simulink model "RL_FA_system_5ESD0"  (R2021b)
settings: Solver=VariableStepAuto  StartTime=0.0  StopTime=10.0  RelTol=1e-3
values from neighbouring files (symbols this model uses):
  b = 1*10.^-5    (= 1e-05)    [condesign.m]    (also in controller.mat)
  d = 3.125*10.^-5    (= 3.125e-05)    [condesign.m]    (also in controller.mat)
  J1 = 5.8198*10.^-6    (= 5.8198e-06)    [condesign.m]    (also in controller.mat)
  J2 = 4.769*10.^-6    (= 4.769e-06)    [condesign.m]    (also in controller.mat)
  k = 0.2656    [condesign.m]    (also in controller.mat)
  Km = 4.4*10.^-2    (= 0.044)    [condesign.m]    (also in controller.mat)
libraries: cstblocks x2
settings Model: Creator=whendrix  LastModifiedBy=s164604
settings SolverCC: AlgebraicLoopSolver=TrustRegion
settings DebuggingCC: SFMachineParentedDataDiag=warning

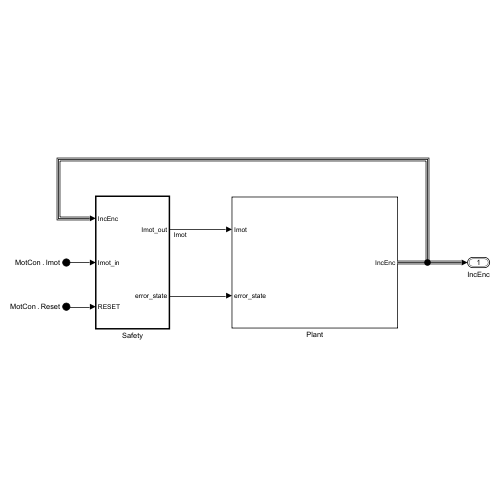
[thumbnail: Simulink's stored preview of the top-level diagram]
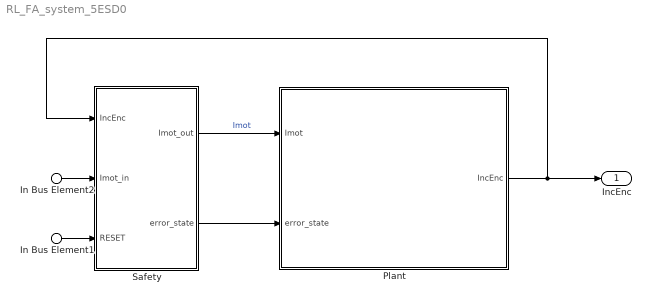
== system RL_FA_system_5ESD0 ==
  In Bus Element2 : Inport  PortName=MotCon  Element=Imot
  In Bus Element1 : Inport  PortName=MotCon  Element=Reset
  Plant : Subsystem
  Safety : Subsystem  TreatAsAtomicUnit=on
  IncEnc : Outport  OutDataTypeStr=Bus: IncEnc
  wires:
  Safety/1(Imot_out) -> Plant/1(Imot)  "Imot"
  In Bus Element2/1 -> Safety/2(Imot_in)
  In Bus Element1/1 -> Safety/3(RESET)
  Plant/1(IncEnc) -> IncEnc/1, Safety/1(IncEnc)
  Safety/2(error_state) -> Plant/2(error_state)

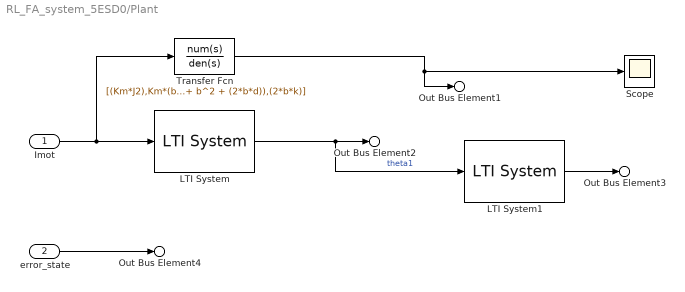
== system RL_FA_system_5ESD0/Plant ==
  Imot : Inport
  error_state : Inport  Port=2
  LTI System : cstblocks/LTI System  sys=G  IC=[]
  LTI System1 : cstblocks/LTI System  sys=G2  IC=[]
  Scope : Scope
  Transfer Fcn : TransferFcn  Numerator=[(Km*J2),Km*(b+d),(Km*k)]  Denominator=[(J1*J2),(J1+J2)*(d+b),((J1+J2)*k + b^2 + (2*b*d)),(2*b*k)]
  Out Bus Element4 : Outport  PortName=IncEnc  Element=error_state
  Out Bus Element2 : Outport  PortName=IncEnc  Element=theta1
  Out Bus Element1 : Outport  PortName=IncEnc  Element=omega1
  Out Bus Element3 : Outport  PortName=IncEnc  Element=theta2
  wires:
  LTI System/1 -> LTI System1/1, Out Bus Element2/1  "theta1"
  LTI System1/1 -> Out Bus Element3/1
  error_state/1 -> Out Bus Element4/1
  Imot/1 -> Transfer Fcn/1, LTI System/1
  Transfer Fcn/1 -> Scope/1, Out Bus Element1/1

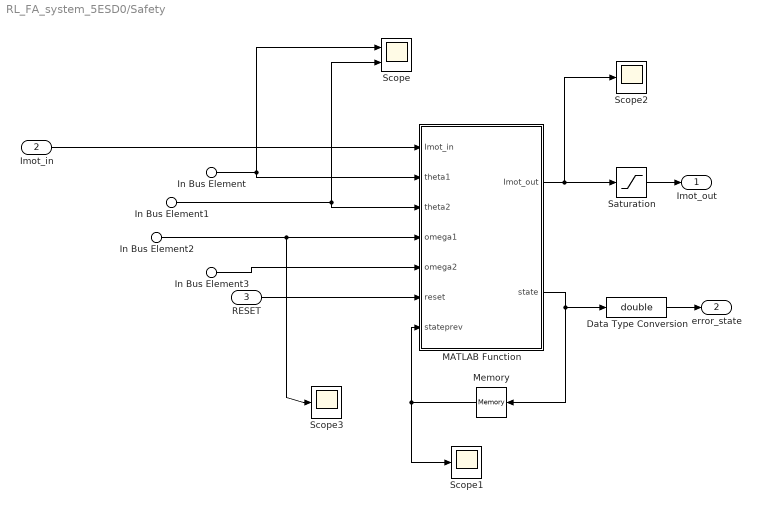
== system RL_FA_system_5ESD0/Safety ==
  In Bus Element : Inport  PortName=IncEnc  Element=theta1
  In Bus Element2 : Inport  PortName=IncEnc  Element=omega1
  In Bus Element1 : Inport  PortName=IncEnc  Element=theta2
  In Bus Element3 : Inport  PortName=IncEnc  Element=omega2
  Imot_in : Inport  Port=2
  RESET : Inport  Port=3
  Data Type Conversion : DataTypeConversion  OutDataTypeStr=double
  MATLAB Function : MATLAB Function  TreatAsAtomicUnit=on
  Memory : Memory
  Saturation : Saturate  UpperLimit=1.83  LowerLimit=-1.83
  Scope : Scope  NumInputPorts=2
  Scope1 : Scope
  Scope2 : Scope
  Scope3 : Scope
  Imot_out : Outport
  error_state : Outport  Port=2
  wires:
  Imot_in/1 -> MATLAB Function/1(Imot_in)
  MATLAB Function/1(Imot_out) -> Scope2/1, Saturation/1
  RESET/1 -> MATLAB Function/6(reset)
  In Bus Element/1 -> Scope/1, MATLAB Function/2(theta1)
  In Bus Element1/1 -> Scope/2, MATLAB Function/3(theta2)
  In Bus Element2/1 -> Scope3/1, MATLAB Function/4(omega1)
  In Bus Element3/1 -> MATLAB Function/5(omega2)
  MATLAB Function/2(state) -> Memory/1, Data Type Conversion/1
  Memory/1 -> Scope1/1, MATLAB Function/7(stateprev)
  Data Type Conversion/1 -> error_state/1
  Saturation/1 -> Imot_out/1

== matlab function RL_FA_system_5ESD0/Safety/MATLAB Function ==
  data: Imot_in input; theta1 input; theta2 input; Imot_out output; omega1 input; omega2 input; reset input; stateprev input; state output
function [Imot_out,state]  = fcn(Imot_in,theta1,theta2,omega1,omega2,reset,stateprev)
%#codegen
omega = max(abs(omega1),abs(omega2));
thetadif = abs(theta1-theta2);
% persistent state;
% 
% if isempty(state)
%     state=0;
% end

state=stateprev;

switch state
    case 0   
        if (omega > 400) || (thetadif > 0.5) %error conditions
         state=1;
         Imot_out=0;
        elseif reset==1
            state=2;
            Imot_out=0;
        else
            state=0;
            Imot_out = Imot_in;
        end
        
    case 1  %error state
        if reset==1
            state=2;
            Imot_out=0;
        else
            state=1;
            Imot_out=0;
        end
        
    case 2
        if reset==0;
            state=0;
            Imot_out=0;
        else
            state=2;
            Imot_out=0;
        end
    otherwise Imot_out=0;
end
